simulink model "ad9361_rx_wlan_testbench"  (R2018b)
settings: Solver=VariableStepAuto  StartTime=0.0  StopTime=0.008500  RelTol=1e-3
model workspace (MAT data in the model file):
  SampleTime_rx = 5e-08
undefined symbols (not defined in the file or in its folder): designMultirateFIR, magnitude
libraries: commsource2 x1, ad9371_utilities x1, dspmlti4 x1, dspmathops x1, ad9361_models x1
CloseFcn:
  | clear SampleTime_rx;
settings Model: PauseTimes=9e-6  Creator=mmohamed  LastModifiedBy=spagadar
settings DataIOCC: InspectSignalLogs=on
settings OptimizationCC: EfficientMapNaN2IntZero=off
settings DebuggingCC: LibraryContextMissingDiagnostic=none
settings HardwareCC: TargetBitPerPointer=64  TargetBitPerSizeT=64  TargetBitPerPtrDiffT=64  TargetLongLongMode=on  TargetIntDivRoundTo=Zero  TargetEndianess=LittleEndian  TargetWordSize=64  TargetHWDeviceType=MATLAB Host  ProdEqTarget=off
settings SFSimCC: SimUseLocalCustomCode=off
settings CodeAppCC: MaxIdLength=128
settings GRTTargetCC: TargetLangStandard=C89/C90 (ANSI)  CombineOutputUpdateFcns=off  GRTInterface=on

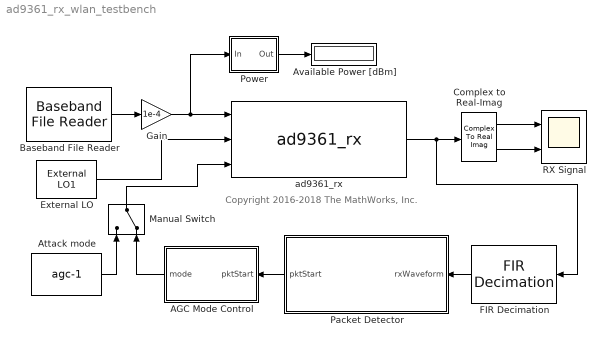
== system ad9361_rx_wlan_testbench ==
  note: Copyright 2016-2018 The MathWorks, Inc.
  AGC Mode Control : MATLAB Function  TreatAsAtomicUnit=on
  Attack mode : Constant  AncestorBlock="ad9361_models/ad9361_rx/Attack  mode"  Value=agc-1  SampleTime=-1  mask{agc=Manual}
      mask prompts: agc "Attack Mode"
      mask TypeOptions agc: Manual | Fast | Slow
      mask DialogControl DescGroupVar Prompt: AGC Attack Mode
      mask Display: disp('AGC Mode')
  Available Power [dBm] : Display
  Baseband File Reader : commsource2/Baseband File Reader  Filename=C:\Users\spagadar\Documents\MATLAB\tuneAD9361AGC\ad9361_rx_input_files\testWaveform_21_Jun_2019_15_03_57.bb  InheritSampleTimeFromFile=on  SampleTime=1  SamplesPerFrame=1  CyclicRepetition=off  FileEndOutputPort=off  SimulateUsing=Code generation
      settings: SourceProductName=Communications System Toolbox  SourceProductBaseCode=CM
  Complex to Real-Imag : ComplexToRealImag
  External LO : ad9371_utilities/External LO1  PN=[-95 -110 -110 -125 -157]  Freq=[1e3 1e4 1e5 1e6 3e6]  PH=Random
      settings: SourceProductName=RF Blockset Models for Analog Devices RF Transceivers  SourceProductBaseCode=SIM_RF_TRANS
  FIR Decimation : dspmlti4/FIR Decimation  FilterSource=Auto  h=designMultirateFIR(1,2)  D=2  filtStruct=Direct form  FilterObject=FDECIM  InputProcessing=Columns as channels (frame based)  framing=Allow multirate processing  inputOffset=0  outputBufInitCond=0  roundingMode=Floor  overflowMode=off  firstCoeffDataTypeStr=Inherit: Same word length as input  firstCoeffMin=[]  firstCoeffMax=[]  firstCoeffLastDataTypeStr=Inherit: Same word length as input  outputDataTypeStr=Inherit: Same as accumulator  outputMin=[]  outputMax=[]  outputLastDataTypeStr=Inherit: Same as accumulator
  Gain : Gain  Gain=1e-4
  Manual Switch : ManualSwitch  CurrentSetting=0
  Packet Detector : MATLAB Function  TreatAsAtomicUnit=on
  Power : Subsystem  mask{R=50}
      mask prompts: R "Reference Impedance [Ohm]"
      mask DialogControl DescGroupVar Prompt: Power Meter
      mask Display: disp('Power \nMeter');
  RX Signal : Scope  NumInputPorts=2
  ad9361_rx : ad9361_models/ad9361_rx  TestSignal=Custom  LO=2.4e9  RF=2.4e9  Trf=SampleTime_rx/2.0  RF_BW=40  IQ_rate=40
      settings: SourceProductName=RF Blockset Models for Analog Devices RF Transceivers  SourceProductBaseCode=SIM_RF_TRANS
  wires:
  ad9361_rx/1 -> Complex to Real-Imag/1, FIR Decimation/1
  Packet Detector/1(pktStart) -> AGC Mode Control/1(pktStart)
  FIR Decimation/1 -> Packet Detector/1(rxWaveform)
  Manual Switch/1 -> ad9361_rx/3
  Gain/1 -> Power/1(In), ad9361_rx/1
  External LO/1 -> ad9361_rx/2
  Baseband File Reader/1 -> Gain/1
  Complex to Real-Imag/1 -> RX Signal/1
  Complex to Real-Imag/2 -> RX Signal/2
  Power/1(Out) -> Available Power [dBm]/1
  Attack mode/1 -> Manual Switch/1
  AGC Mode Control/1(mode) -> Manual Switch/2

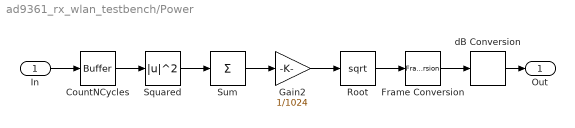
== system ad9361_rx_wlan_testbench/Power ==
  In : Inport
  CountNCycles : Buffer  N=1024
  Frame Conversion : FrameConversion  OutFrame=Sample-based
  Gain2 : Gain  Gain=1/1024
  Root : Sqrt  SaturateOnIntegerOverflow=on
  Squared : Math  Operator=magnitude^2  SaturateOnIntegerOverflow=on
  Sum : Sum  Inputs=+  CollapseMode=Specified dimension
  dB Conversion : dspmathops/dB Conversion  dBtype=dBm  intype=Amplitude  R=R  fuzz=on
      settings: SourceProductName=DSP System Toolbox
  Out : Outport
  wires:
  dB Conversion/1 -> Out/1
  In/1 -> CountNCycles/1
  Frame Conversion/1 -> dB Conversion/1
  CountNCycles/1 -> Squared/1
  Squared/1 -> Sum/1
  Sum/1 -> Gain2/1
  Root/1 -> Frame Conversion/1
  Gain2/1 -> Root/1

== matlab function ad9361_rx_wlan_testbench/AGC Mode Control ==
  data: mode output; pktStart input
function mode = fcn(pktStart)

persistent prev;
if isempty(prev)
    prev = 0;
    mode = 0;
end

if (pktStart == 0)
    prev = 0;
    lstf_sample_count = 0;
    mode = 0;
else
    lstf_sample_count = prev + pktStart;
    if ((lstf_sample_count >= 1) && (lstf_sample_count <= 80))
        prev = lstf_sample_count;
        mode = 1;
    else
        prev = -10000;
        mode = 0;
    end   
end

== matlab function ad9361_rx_wlan_testbench/Packet Detector ==
  data: pktStart output; rxWaveform input
function pktStart = fcn(rxWaveform)

% Packet detect and determine coarse packet offset
persistent buffer;
persistent count;
if isempty(count)
    count = 0;
    buffer = zeros(160, 1)+1i*zeros(160, 1);
    buffer(1) = rxWaveform;
else
    count = count+1;
    buffer = circshift(buffer, 1);
    buffer(1) = rxWaveform;
end
pktOffset = wlanPacketDetect(buffer,'CBW20');

if isempty(pktOffset)
  % No packet detected
  pktStart = false;  
else
  % Packet detected
  pktStart = true;  
end
